simulink library "desat_controller_lib"  (R2018b)
settings: Solver=VariableStepAuto  StartTime=0.0  StopTime=10.0  RelTol=1e-3
undefined symbols (not defined in the file or in its folder): fswParams
libraries: vrlib x2, dspmtrx3 x2, two_norm x1
settings Model: Creator=sophiakim  LastModifiedBy=Nick's PC

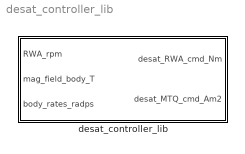
== system desat_controller_lib ==
  desat_controller_lib : Subsystem

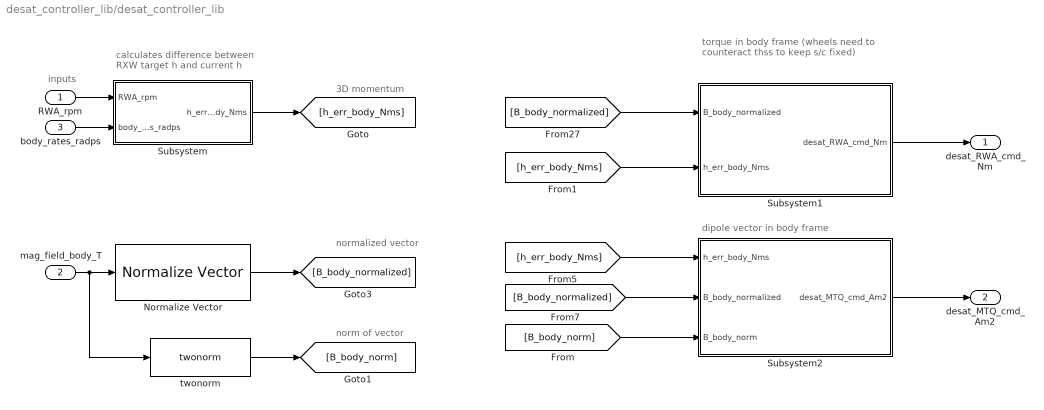
== system desat_controller_lib/desat_controller_lib ==
  note: norm of vector
  note: normalized vector
  note: torque in body frame (wheels need to
      | counteract thss to keep s/c fixed)
  note: dipole vector in body frame
  note: calculates difference between
      | RXW target h and current h
  note: inputs
  note: 3D momentum
  RWA_rpm : Inport
  mag_field_body_T : Inport  Port=2
  body_rates_radps : Inport  Port=3
  Normalize Vector : vrlib/Utilities/Normalize Vector  maxzero=0
      settings: SourceProductName=Simulink 3D Animation  SourceProductBaseCode=VR
  Subsystem : Subsystem
  Subsystem1 : Subsystem
  Subsystem2 : Subsystem
  twonorm : two_norm/twonorm  SystemSampleTime=-1
  desat_RWA_cmd_Nm : Outport
  "desat_MTQ_cmd_Am2 " : Outport  Port=2
  wires:
  mag_field_body_T/1 -> twonorm/1, Normalize Vector/1
  Normalize Vector/1 -> [B_body_normalized]
  RWA_rpm/1 -> Subsystem/1(RWA_rpm)
  Subsystem/1(h_err_body_Nms) -> [h_err_body_Nms]
  [B_body_normalized] -> Subsystem1/1("B_body_normalized ")
  [h_err_body_Nms] -> Subsystem1/2(h_err_body_Nms)
  Subsystem1/1(desat_RWA_cmd_Nm) -> desat_RWA_cmd_Nm/1
  [h_err_body_Nms] -> Subsystem2/1(h_err_body_Nms)
  [B_body_normalized] -> Subsystem2/2(B_body_normalized)
  twonorm/1 -> [B_body_norm]
  Subsystem2/1(desat_MTQ_cmd_Am2) -> "desat_MTQ_cmd_Am2 "/1
  [B_body_norm] -> Subsystem2/3(B_body_norm)
  body_rates_radps/1 -> Subsystem/2("body_rates_radps ")

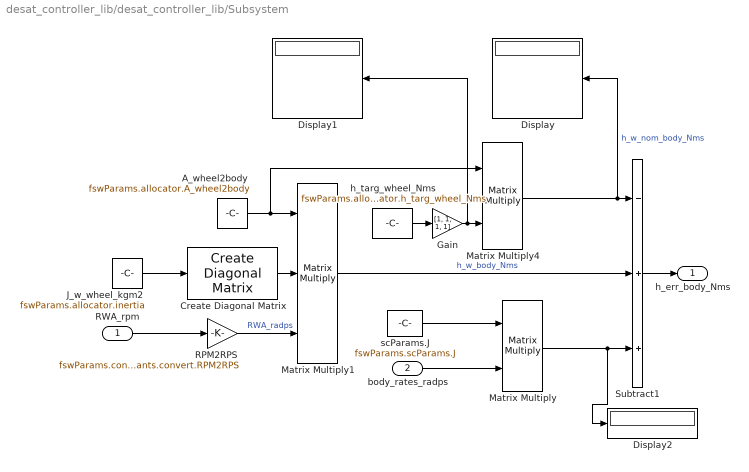
== system desat_controller_lib/desat_controller_lib/Subsystem ==
  RWA_rpm : Inport
  "body_rates_radps " : Inport  Port=2
  "A_wheel2body " : Constant  Value=fswParams.allocator.A_wheel2body
  Create Diagonal Matrix : dspmtrx3/Create Diagonal Matrix
      settings: SourceProductName=DSP System Toolbox  SourceProductBaseCode=DS
  Display : Display
  Display1 : Display
  Display2 : Display
  Gain : Gain  Gain=[1, 1, 1, 1]
  J_w_wheel_kgm2 : Constant  Value=fswParams.allocator.inertia
  Matrix Multiply : Product  Multiplication=Matrix(*)
  Matrix Multiply1 : Product  Inputs=3  Multiplication=Matrix(*)
  Matrix Multiply4 : Product  Multiplication=Matrix(*)
  RPM2RPS : Gain  Gain=fswParams.constants.convert.RPM2RPS
  Subtract1 : Sum  Inputs=-++
  h_targ_wheel_Nms : Constant  Value=fswParams.allocator.h_targ_wheel_Nms
  "scParams.J " : Constant  Value=fswParams.scParams.J
  h_err_body_Nms : Outport
  wires:
  RWA_rpm/1 -> RPM2RPS/1
  Subtract1/1 -> h_err_body_Nms/1
  J_w_wheel_kgm2/1 -> Create Diagonal Matrix/1
  "A_wheel2body "/1 -> Matrix Multiply4/1, Matrix Multiply1/1
  Matrix Multiply4/1 -> Display/1, Subtract1/1  "h_w_nom_body_Nms"
  Matrix Multiply1/1 -> Subtract1/2  "h_w_body_Nms"
  h_targ_wheel_Nms/1 -> Gain/1
  RPM2RPS/1 -> Matrix Multiply1/3  "RWA_radps"
  Create Diagonal Matrix/1 -> Matrix Multiply1/2
  Gain/1 -> Display1/1, Matrix Multiply4/2
  Matrix Multiply/1 -> Display2/1, Subtract1/3
  "scParams.J "/1 -> Matrix Multiply/1
  "body_rates_radps "/1 -> Matrix Multiply/2

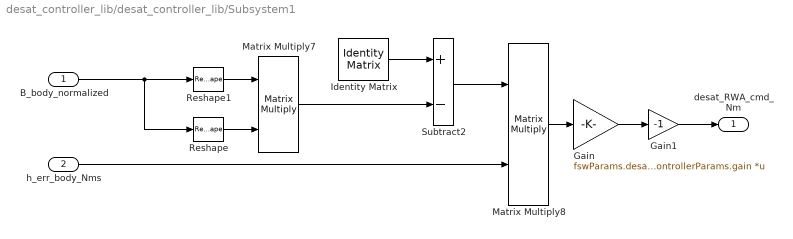
== system desat_controller_lib/desat_controller_lib/Subsystem1 ==
  "B_body_normalized " : Inport
  h_err_body_Nms : Inport  Port=2
  Gain : Gain  Gain=fswParams.desatcontrollerParams.gain  Multiplication=Matrix(K*u) (u vector)
  Gain1 : Gain  Gain=-1
  Identity Matrix : dspmtrx3/Identity Matrix  Inherit=off  N=3  Ts=inf  dataType=double  isSigned=on  wordLen=16  udDataType=sfix(16)  fracBitsMode=Best precision  numFracBits=15  OutDataTypeStr=double  LastOutDataTypeStr=double
      settings: SourceProductName=DSP System Toolbox
  Matrix Multiply7 : Product  Multiplication=Matrix(*)
  Matrix Multiply8 : Product  Multiplication=Matrix(*)
  Reshape : Reshape  OutputDimensionality=Row vector (2-D)
  Reshape1 : Reshape  OutputDimensionality=Column vector (2-D)
  Subtract2 : Sum  Inputs=+-
  desat_RWA_cmd_Nm : Outport
  wires:
  Reshape/1 -> Matrix Multiply7/2
  Matrix Multiply7/1 -> Subtract2/2
  h_err_body_Nms/1 -> Matrix Multiply8/2
  Identity Matrix/1 -> Subtract2/1
  Reshape1/1 -> Matrix Multiply7/1
  "B_body_normalized "/1 -> Reshape/1, Reshape1/1
  Gain1/1 -> desat_RWA_cmd_Nm/1
  Matrix Multiply8/1 -> Gain/1
  Subtract2/1 -> Matrix Multiply8/1
  Gain/1 -> Gain1/1

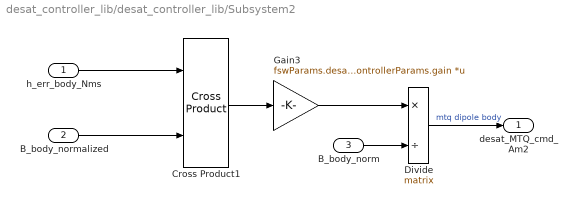
== system desat_controller_lib/desat_controller_lib/Subsystem2 ==
  h_err_body_Nms : Inport
  B_body_normalized : Inport  Port=2
  B_body_norm : Inport  Port=3
  Cross Product1 : vrlib/Utilities/Cross Product
      settings: SourceProductBaseCode=VR
  Divide : Product  Inputs=*/  Multiplication=Matrix(*)
  Gain3 : Gain  Gain=fswParams.desatcontrollerParams.gain  Multiplication=Matrix(K*u) (u vector)
  desat_MTQ_cmd_Am2 : Outport
  wires:
  B_body_normalized/1 -> Cross Product1/2
  h_err_body_Nms/1 -> Cross Product1/1
  Cross Product1/1 -> Gain3/1
  Gain3/1 -> Divide/1
  B_body_norm/1 -> Divide/2
  Divide/1 -> desat_MTQ_cmd_Am2/1  "mtq dipole body"
